simulink library "tire"  (R2020b)
settings: Solver=VariableStepAuto  StartTime=0.0  StopTime=10.0  RelTol=1e-3
undefined symbols (not defined in the file): Brakes_caliperD, Brakes_effectiveR, Brakes_kineticMu, Brakes_pads_front, Brakes_staticMu, Rim_mass, Tire_Cg, Tire_Cx, Tire_Cy, Tire_Lx, Tire_Ly, Tire_mass, Tire_muMax, Tire_muMin, Tire_prs_front, Tire_radius, Tire_VerticalK, Wheel_inertia, Wheel_width, X, Y, Z
libraries: nesl_utility x26, sm_lib x22, vehdynlibtire x2
(part 3 of 3)

== matlab function tire/Wheel - Fiala/w - Wheel to Tire transform ==
  data: IA input; u input; y output; sideSign parameter
function y = fcn(IA,u,sideSign)
 
y=[1 0 0;0 cos(-IA*sideSign) -sin(-IA*sideSign);0 sin(-IA*sideSign) cos(-IA*sideSign)]*u;

== matlab function tire/Wheel - Fiala/Camber ==
  data: R input; IA output; sideSign parameter
function IA = fcn(R,sideSign)
IA = -acos(R(3,3))*sideSign*sign(R(3,2));

== matlab function tire/Wheel - Fiala/F - Tire to Wheel transform ==
  data: IA input; u input; y output; sideSign parameter
function y = fcn(IA,u,sideSign)
 
y=[1 0 0;0 cos(IA*sideSign) -sin(IA*sideSign);0 sin(IA*sideSign) cos(IA*sideSign)]*u;

== matlab function tire/Wheel - Fiala/M - Tire to Wheel transform ==
  data: IA input; u input; y output; sideSign parameter
function y = fcn(IA,u,sideSign)
 
y=[1 0 0;0 cos(IA*sideSign) -sin(IA*sideSign);0 sin(IA*sideSign) cos(IA*sideSign)]*u;

== matlab function tire/Wheel - Combined Slip/Camber ==
  data: R input; IA output; sideSign parameter
function IA = fcn(R,sideSign)
IA = acos(R(3,3))*sideSign*sign(R(2,3));

== matlab function tire/Wheel - Combined Slip/F - Tire to Wheel transform ==
  data: IA input; u input; y output; sideSign parameter
function y = fcn(IA,u,sideSign)
 
y=[1 0 0;0 cos(IA*sideSign) -sin(IA*sideSign);0 sin(IA*sideSign) cos(IA*sideSign)]*u;

== matlab function tire/Wheel - Combined Slip/M - Tire to Wheel transform ==
  data: IA input; u input; y output; sideSign parameter
function y = fcn(IA,u,sideSign)
 
y=[1 0 0;0 cos(IA*sideSign) -sin(IA*sideSign);0 sin(IA*sideSign) cos(IA*sideSign)]*u;

== matlab function tire/Wheel - Combined Slip/Toe ==
  data: R input; toe output
function toe = fcn(R)
toe = acos(R(1,1))*sign(R(2,1));

== matlab function tire/Wheel - Combined Slip/V - Wheel to Tire transform ==
  data: IA input; u input; y output; sideSign parameter
function y = fcn(IA,u,sideSign)
 
y=[1 0 0;0 cos(-IA*sideSign) -sin(-IA*sideSign);0 sin(-IA*sideSign) cos(-IA*sideSign)]*u;

== matlab function tire/Wheel - Fiala/Toe ==
  data: R input; toe output
function toe = fcn(R)
toe = acos(R(1,1))*sign(R(2,1));

== matlab function tire/Wheel - Combined Slip/w - Wheel to Tire transform ==
  data: IA input; u input; y output; sideSign parameter
function y = fcn(IA,u,sideSign)
 
y=[1 0 0;0 cos(-IA*sideSign) -sin(-IA*sideSign);0 sin(-IA*sideSign) cos(-IA*sideSign)]*u;

== matlab function tire/Wheel - Fiala/V - Wheel to Tire transform ==
  data: IA input; u input; y output; sideSign parameter
function y = fcn(IA,u,sideSign)
 
y=[1 0 0;0 cos(-IA*sideSign) -sin(-IA*sideSign);0 sin(-IA*sideSign) cos(-IA*sideSign)]*u;
